simulink subsystem "cvrs_ventricle_contractility"  (R2019b)
settings: Solver=VariableStepAuto  StartTime=0.0  StopTime=10.0  RelTol=1e-3
settings Model: Creator=RH  LastModifiedBy=RH

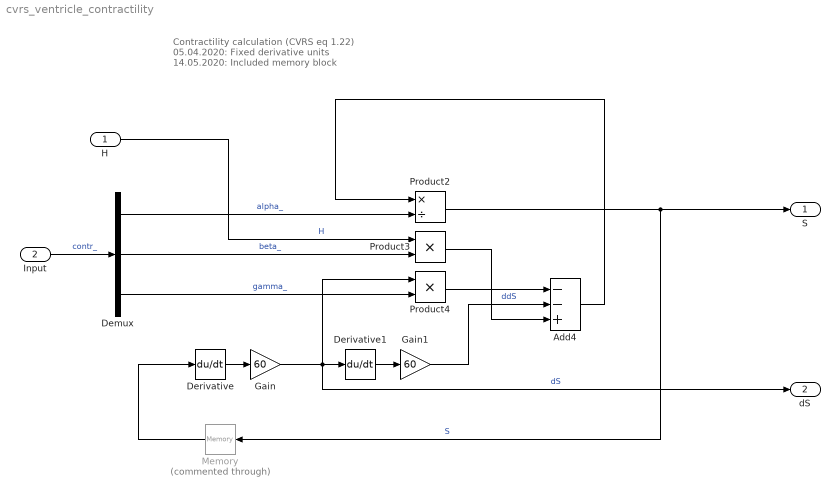
== system cvrs_ventricle_contractility ==
  note: Contractility calculation
      | (CVRS eq 1.22)
      | 05.04.2020: Fixed derivative units
      | 14.05.2020: Included memory block
  H : Inport  Unit=1/min
  Input : Inport  Port=2  PortDimensions=3
  Add4 : Sum  Inputs=--+
  Demux : Demux  Outputs=3
  Derivative : Derivative
  Derivative1 : Derivative
  Gain : Gain  Gain=60
  Gain1 : Gain  Gain=60
  Memory : Memory  Commented=through
  Product2 : Product  Inputs=*/
  Product3 : Product  Inputs=**
  Product4 : Product  Inputs=**
  S : Outport  Unit=mmHg
  dS : Outport  Port=2  Unit=mmHg/min
  wires:
  H/1 -> Product3/1  "H"
  Demux/3 -> Product4/2  "gamma_"
  Demux/1 -> Product2/2  "alpha_"
  Demux/2 -> Product3/2  "beta_"
  Product2/1 -> Memory/1, S/1  "S"
  Product4/1 -> Add4/1
  Derivative1/1 -> Gain1/1
  Add4/1 -> Product2/1
  Product3/1 -> Add4/3
  Derivative/1 -> Gain/1
  Gain/1 -> Product4/1, Derivative1/1, dS/1  "dS"
  Gain1/1 -> Add4/2  "ddS"
  Memory/1 -> Derivative/1
  Input/1 -> Demux/1  "contr_"
